simulink model "problem3"  (R2020a)
settings: Solver=VariableStepAuto  StartTime=0.0  StopTime=10.0  RelTol=1e-3
settings Model: Creator=HP  LastModifiedBy=HP

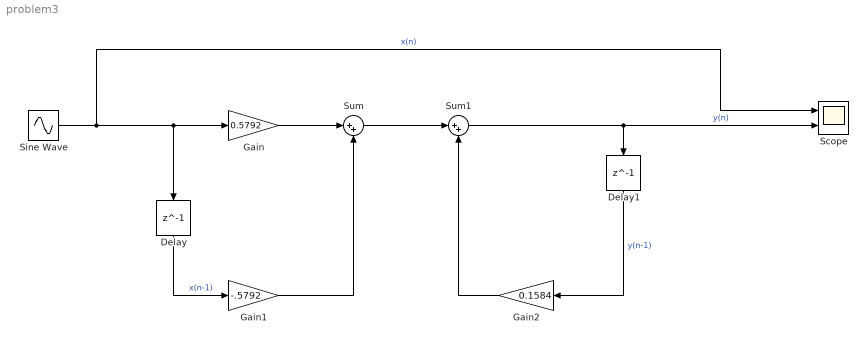
== system problem3 ==
  Delay : Delay  DelayLength=1  InitialCondition=0
  Delay1 : Delay  DelayLength=1  InitialCondition=0
  Gain : Gain  Gain=0.5792
  Gain1 : Gain  Gain=-.5792
  Gain2 : Gain  Gain=0.1584
  Scope : Scope  NumInputPorts=2
  Sine Wave : Sin  SampleTime=0
  Sum : Sum  Inputs=|++
  Sum1 : Sum  Inputs=|++
  wires:
  Delay/1 -> Gain1/1  "x(n-1)"
  Gain/1 -> Sum/1
  Gain1/1 -> Sum/2
  Sum/1 -> Sum1/1
  Gain2/1 -> Sum1/2
  Sum1/1 -> Delay1/1, Scope/2  "y(n)"
  Delay1/1 -> Gain2/1  "y(n-1)"
  Sine Wave/1 -> Scope/1, Gain/1, Delay/1  "x(n)"
